simulink model "Noise_shaping_block"  (R2012b)
settings: Solver=ode45  StartTime=0.0  StopTime=10.0  RelTol=1e-3
settings Model: Creator=ayush  LastModifiedBy=ayush

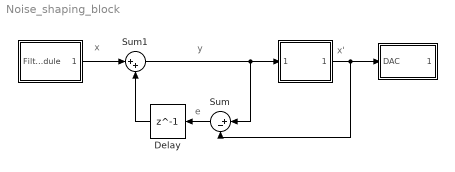
== system Noise_shaping_block ==
  note: x'
  note: e
  note: y
  note: x
  " " : Subsystem
  "  " : Subsystem
  "   " : Subsystem
  Delay : Delay  DelayLength=1  InitialCondition=0
  Sum : Sum  Inputs=|+-
  Sum1 : Sum  Inputs=|++
  wires:
  "  "/1(" ") -> " "/1("\t\t\t\t\tDAC"), Sum/2
  Sum1/1 -> "  "/1(Quantizer), Sum/1
  Sum/1 -> Delay/1
  Delay/1 -> Sum1/2
  "   "/1("  ") -> Sum1/1

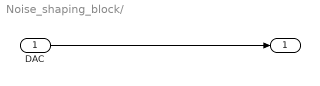
== system Noise_shaping_block/  ==
  "\t\t\t\t\tDAC" : Inport
  "  " : Outport
  wires:
  "\t\t\t\t\tDAC"/1 -> "  "/1

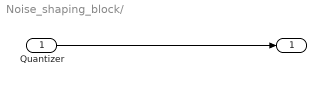
== system Noise_shaping_block/   ==
  Quantizer : Inport
  " " : Outport
  wires:
  Quantizer/1 -> " "/1

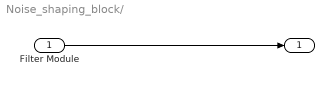
== system Noise_shaping_block/    ==
  Filter Module : Inport
  "  " : Outport
  wires:
  Filter Module/1 -> "  "/1
